simulink model "motor_simu3"  (R2012b)
settings: Solver=ode45  StartTime=0.0  StopTime=500
undefined symbols (not defined in the file or in its folder): Jc, Jri
libraries: simulink x2
settings Model: Creator=Felipe  LastModifiedBy=NSEE
settings DataIOCC: SignalLoggingSaveFormat=ModelDataLogs
settings DebuggingCC: FcnCallInpInsideContextMsg=UseLocalSettings
settings GRTTargetCC: CombineOutputUpdateFcns=off  GRTInterface=on

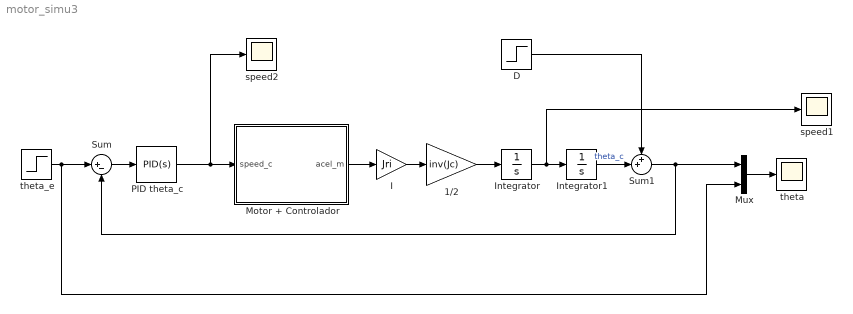
== system motor_simu3 ==
  1/2 : Gain  Gain=inv(Jc)
  D : Step  Time=350  After=(pi/4)/10  SampleTime=0
  I : Gain  Gain=Jri
  Integrator : Integrator
  Integrator1 : Integrator
  Motor + Controlador : Subsystem
  Mux : Mux  Inputs=2
  PID theta_c : simulink/Continuous/PID Controller  Controller=PID  TimeDomain=Continuous-time  SampleTime=1  IntegratorMethod=Forward Euler  FilterMethod=Forward Euler  Form=Parallel  P=1.50145105035343  I=0.01  D=-36.2038912896366  N=0.0414720903435931  InitialConditionSource=internal  InitialConditionForIntegrator=0  InitialConditionForFilter=0  ExternalReset=none  LimitOutput=off  UpperSaturationLimit=inf  LowerSaturationLimit=-inf  LinearizeAsGain=off  AntiWindupMode=none  Kb=1  TrackingMode=off  Kt=1  PParamMin=[]  PParamMax=[]  IParamMin=[]  IParamMax=[]  DParamMin=[]  DParamMax=[]  NParamMin=[]  NParamMax=[]  KbParamMin=[]  KbParamMax=[]  KtParamMin=[]  KtParamMax=[]  POutMin=[]  POutMax=[]  IOutMin=[]  IOutMax=[]  DOutMin=[]  DOutMax=[]  NOutMin=[]  NOutMax=[]  KbOutMin=[]  KbOutMax=[]  KtOutMin=[]  KtOutMax=[]  IntegratorOutMin=[]  IntegratorOutMax=[]  FilterOutMin=[]  FilterOutMax=[]  SumOutMin=[]  SumOutMax=[]  SumI1OutMin=[]  SumI1OutMax=[]  SumI2OutMin=[]  SumI2OutMax=[]  SumI3OutMin=[]  SumI3OutMax=[]  SumDOutMin=[]  SumDOutMax=[]  SaturationOutMin=[]  SaturationOutMax=[]  IntegratorContinuousStateAttributes=''  IntegratorStateMustResolveToSignalObject=off  IntegratorRTWStateStorageClass=Auto  FilterContinuousStateAttributes=''  FilterStateMustResolveToSignalObject=off  FilterRTWStateStorageClass=Auto
  Sum : Sum  Inputs=|+-
  Sum1 : Sum  Inputs=++|
  speed1 : Scope
      settings: SaveName=ScopeData3
  speed2 : Scope
      settings: SaveName=ScopeData4
  theta : Scope
      settings: YMin=1.5  YMax=5.75
  theta_e : Step  After=(pi)  SampleTime=0
  wires:
  Motor + Controlador/1(acel_m) -> I/1
  I/1 -> 1/2/1
  Integrator/1 -> Integrator1/1, speed1/1
  PID theta_c/1 -> speed2/1, Motor + Controlador/1(speed_c)
  theta_e/1 -> Sum/1, Mux/2
  Sum/1 -> PID theta_c/1
  Mux/1 -> theta/1
  1/2/1 -> Integrator/1
  Integrator1/1 -> Sum1/2  "theta_c"
  D/1 -> Sum1/1
  Sum1/1 -> Sum/2, Mux/1

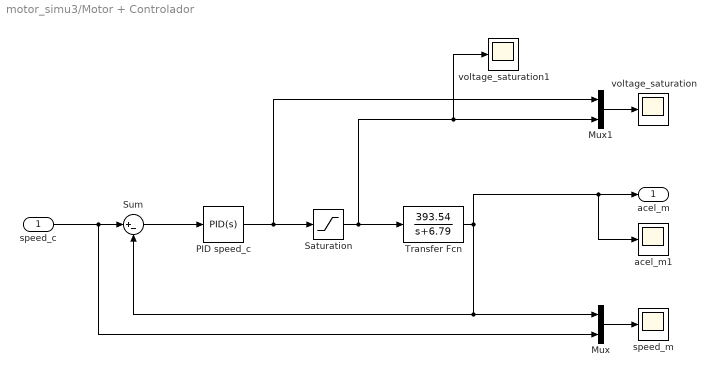
== system motor_simu3/Motor + Controlador ==
  speed_c : Inport
  Mux : Mux  Inputs=2
  Mux1 : Mux  Inputs=2
  PID speed_c : simulink/Continuous/PID Controller  Controller=PID  TimeDomain=Continuous-time  SampleTime=1  IntegratorMethod=Forward Euler  FilterMethod=Forward Euler  Form=Parallel  P=0.0702810444210293  I=0.641986943674692  D=-0.00114121759053741  N=61.5842631622364  InitialConditionSource=internal  InitialConditionForIntegrator=0  InitialConditionForFilter=0  ExternalReset=none  LimitOutput=off  UpperSaturationLimit=inf  LowerSaturationLimit=-inf  LinearizeAsGain=off  AntiWindupMode=none  Kb=1  TrackingMode=off  Kt=1  PParamMin=[]  PParamMax=[]  IParamMin=[]  IParamMax=[]  DParamMin=[]  DParamMax=[]  NParamMin=[]  NParamMax=[]  KbParamMin=[]  KbParamMax=[]  KtParamMin=[]  KtParamMax=[]  POutMin=[]  POutMax=[]  IOutMin=[]  IOutMax=[]  DOutMin=[]  DOutMax=[]  NOutMin=[]  NOutMax=[]  KbOutMin=[]  KbOutMax=[]  KtOutMin=[]  KtOutMax=[]  IntegratorOutMin=[]  IntegratorOutMax=[]  FilterOutMin=[]  FilterOutMax=[]  SumOutMin=[]  SumOutMax=[]  SumI1OutMin=[]  SumI1OutMax=[]  SumI2OutMin=[]  SumI2OutMax=[]  SumI3OutMin=[]  SumI3OutMax=[]  SumDOutMin=[]  SumDOutMax=[]  SaturationOutMin=[]  SaturationOutMax=[]  IntegratorContinuousStateAttributes=''  IntegratorStateMustResolveToSignalObject=off  IntegratorRTWStateStorageClass=Auto  FilterContinuousStateAttributes=''  FilterStateMustResolveToSignalObject=off  FilterRTWStateStorageClass=Auto
  Saturation : Saturate  UpperLimit=12  LowerLimit=-12
  Sum : Sum  Inputs=|+-
  Transfer Fcn : TransferFcn  Numerator=[393.54]  Denominator=[1 6.79]
  acel_m1 : Scope
      settings: YMin=-0.095  YMax=0
  speed_m : Scope
      settings: YMin=-1e+06  YMax=6e+06  SaveName=ScopeData2
  voltage_saturation : Scope
      settings: YMin=0  YMax=5.25e+06  SaveName=ScopeData5
  voltage_saturation1 : Scope
      settings: TimeRange=500  YMin=-12.5  YMax=12.5  SaveName=ScopeData6
  acel_m : Outport
  wires:
  Saturation/1 -> Transfer Fcn/1, voltage_saturation1/1, Mux1/2
  PID speed_c/1 -> Saturation/1, Mux1/1
  Sum/1 -> PID speed_c/1
  speed_c/1 -> Sum/1, Mux/2
  Transfer Fcn/1 -> acel_m/1, acel_m1/1, Mux/1, Sum/2
  Mux/1 -> speed_m/1
  Mux1/1 -> voltage_saturation/1
